simulink model "s0227"  (Simulink 6.0)
settings: Solver=ode5  SolverMode=SingleTasking  StartTime=0.0  StopTime=10  FixedStep=.1  MaxStep=.1  RelTol=1e-3  AbsTol=1e-6
settings Model: LastModifiedBy=Froriep
settings DataIOCC: LimitDataPoints=off  SaveOutput=off  SaveTime=off
settings OptimizationCC: BooleanDataType=off
settings DebuggingCC: SolverPrmCheckMsg=none
settings HardwareCC: TargetUnknown=on
settings GRTTargetCC: ModelReferenceCompliant=off  MatFileLogging=off

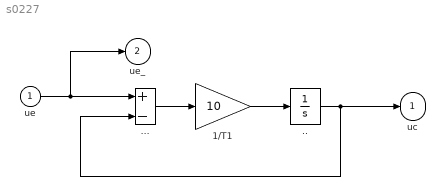
== system s0227 ==
  ue : Inport  Port=1  LatchInput=off
  .. : Integrator  InitialCondition=1.e-6
  ... : Sum  Inputs=+-  SaturateOnIntegerOverflow=on  InputSameDT=on
  1/T1 : Gain  Gain=10  SaturateOnIntegerOverflow=on
  uc : Outport
  ue_ : Outport  Port=2
  wires:
  ../1 -> .../2, uc/1
  ue/1 -> .../1, ue_/1
  1/T1/1 -> ../1
  .../1 -> 1/T1/1
